simulink model "TwoLinkPlanarRobotHybridControl_gen2nomfiles"  (Simulink 9.0)
settings: Solver=ode1  StartTime=0.0  StopTime=10.0  FixedStep=0.01  RelTol=1e-3  EnableMultiTasking=on
values from neighbouring files (symbols this model uses):
  m = [1 1]    [FurutaPendulum_Dynamics.m]    (also in Question_2.m = [m_1 m_2]; test_ForwardDynamics.m = [1 1 1]; test_TwoLinkPlanarRobotDynamics.m = [m1 m2]; test_TwoLinkPlanarRobotHybridControl.m = [m1 m2])
  N = 5    [createEllipsoid.m]
  s = tf('s')    [Current_loop_bode.m]    (also in Question_1.m = 15)
  X = cos(0:2*pi/n:2*pi)    [createCylinder.m]
  Y = sin(0:2*pi/n:2*pi)    [createCylinder.m]
undefined symbols (not defined in the file or in its folder): Z
libraries: sm_lib x13, nesl_utility x9, simulink x1
settings Model: Creator=leavesdown_admin  LastModifiedBy=leavesdown
settings DataIOCC: LimitDataPoints=on  SignalLoggingSaveFormat=ModelDataLogs
settings OptimizationCC: ExpressionDepthLimit=2147483647
settings DebuggingCC: SolverPrmCheckMsg=warning  FcnCallInpInsideContextMsg=warning  StateNameClashWarn=warning
settings GRTTargetCC: GeneratePreprocessorConditionals=Disable all
settings SimscapeCC: SimscapeNormalizeSystem=off
settings ConfigurationSet: Description=SimMechanics 2G

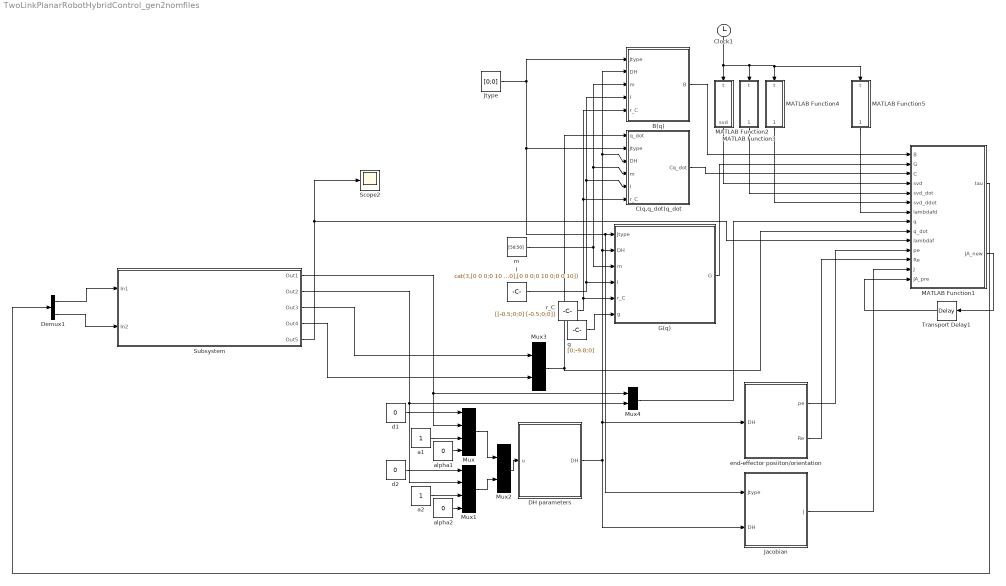
== system TwoLinkPlanarRobotHybridControl_gen2nomfiles ==
  B(q) : MATLAB Function  TreatAsAtomicUnit=on
  C(q,q_dot)q_dot : MATLAB Function  TreatAsAtomicUnit=on
  Clock1 : Clock
  DH parameters : MATLAB Function  TreatAsAtomicUnit=on
  Demux1 : Demux  Outputs=2
  G(q) : MATLAB Function  TreatAsAtomicUnit=on
  I : Constant  Value=cat(3,[0 0 0;0 10 0;0 0 10],[0 0 0;0 10 0;0 0 10])
  Jacobian : MATLAB Function  TreatAsAtomicUnit=on
  Jtype : Constant  Value=[0;0]
  MATLAB Function1 : MATLAB Function  TreatAsAtomicUnit=on
  MATLAB Function2 : MATLAB Function  TreatAsAtomicUnit=on
  MATLAB Function3 : MATLAB Function  TreatAsAtomicUnit=on
  MATLAB Function4 : MATLAB Function  TreatAsAtomicUnit=on
  MATLAB Function5 : MATLAB Function  TreatAsAtomicUnit=on
  Mux : Mux
  Mux1 : Mux
  Mux2 : Mux  Inputs=2
  Mux3 : Mux  Inputs=2
  Mux4 : Mux  Inputs=2
  Scope2 : Scope
  Subsystem : Subsystem
  Transport Delay1 : TransportDelay  DelayTime=0.01
  a1 : Constant
  a2 : Constant
  alpha1 : Constant  Value=0
  alpha2 : Constant  Value=0
  d1 : Constant  Value=0
  d2 : Constant  Value=0
  end-effector posiiton/orientation : MATLAB Function  TreatAsAtomicUnit=on
  g : Constant  Value=[0;-9.8;0]
  m : Constant  Value=[50;50]
  r_C : Constant  Value=[[-0.5;0;0] [-0.5;0;0]]
  wires:
  Subsystem/3(Out3) -> Mux3/1
  Demux1/2 -> Subsystem/2(In2)
  Subsystem/2(Out2) -> Mux4/2, Mux1/2
  Subsystem/4(Out4) -> Mux3/2
  Mux2/1 -> DH parameters/1(u)
  Mux3/1 -> MATLAB Function1/9(q_dot), C(q,q_dot)q_dot/1(q_dot)
  MATLAB Function4/1(svd_ddot) -> MATLAB Function1/6(svd_ddot)
  MATLAB Function3/1(svd_dot) -> MATLAB Function1/5(svd_dot)
  Mux1/1 -> Mux2/2
  m/1 -> B(q)/3(m), C(q,q_dot)q_dot/4(m), G(q)/3(m)
  Mux/1 -> Mux2/1
  MATLAB Function1/2(JA_new) -> Transport Delay1/1
  d1/1 -> Mux/1
  C(q,q_dot)q_dot/1(Cq_dot) -> MATLAB Function1/3(C)
  MATLAB Function2/1(svd) -> MATLAB Function1/4(svd)
  Jtype/1 -> B(q)/1(Jtype), C(q,q_dot)q_dot/2(Jtype), Jacobian/1(Jtype), G(q)/1(Jtype)
  alpha1/1 -> Mux/4
  G(q)/1(G) -> MATLAB Function1/2(G)
  a1/1 -> Mux/3
  alpha2/1 -> Mux1/4
  a2/1 -> Mux1/3
  r_C/1 -> B(q)/5(r_C), C(q,q_dot)q_dot/6(r_C), G(q)/5(r_C)
  Subsystem/1(Out1) -> Mux4/1, Mux/2
  B(q)/1(B) -> MATLAB Function1/1(B)
  Clock1/1 -> MATLAB Function5/1(t), MATLAB Function4/1(t), MATLAB Function3/1(t), MATLAB Function2/1(t)
  Demux1/1 -> Subsystem/1(In1)
  d2/1 -> Mux1/1
  g/1 -> G(q)/6(g)
  MATLAB Function1/1(tau) -> Demux1/1
  I/1 -> B(q)/4(I), C(q,q_dot)q_dot/5(I), G(q)/4(I)
  DH parameters/1(DH) -> Jacobian/2(DH), end-effector posiiton/orientation/1(DH), C(q,q_dot)q_dot/3(DH), B(q)/2(DH), G(q)/2(DH)
  Mux4/1 -> MATLAB Function1/8(q)
  Subsystem/5(Out5) -> MATLAB Function1/10(lambdaf), Scope2/1
  MATLAB Function5/1(lambdafd) -> MATLAB Function1/7(lambdafd)
  Jacobian/1(J) -> MATLAB Function1/13(J)
  Transport Delay1/1 -> MATLAB Function1/14(JA_pre)
  end-effector posiiton/orientation/1(pe) -> MATLAB Function1/11(pe)
  end-effector posiiton/orientation/2(Re) -> MATLAB Function1/12(Re)

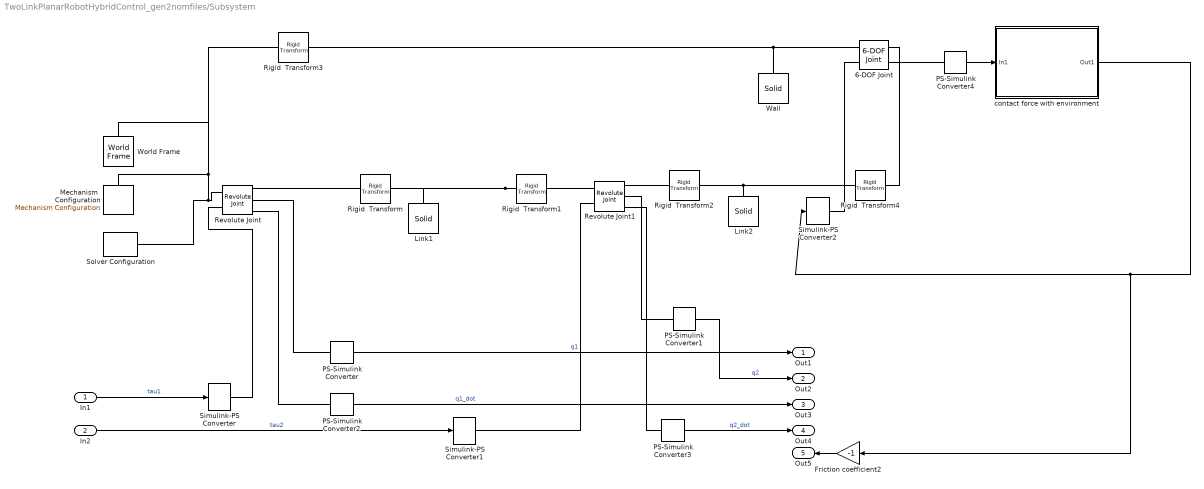
== system TwoLinkPlanarRobotHybridControl_gen2nomfiles/Subsystem ==
  In1 : Inport
  In2 : Inport  Port=2
  6-DOF Joint : sm_lib/Joints/6-DOF Joint  SenseConstraintForce=off  SenseConstraintForceX=off  SenseConstraintForceY=off  SenseConstraintForceZ=off  SenseConstraintTorque=off  SenseConstraintTorqueX=off  SenseConstraintTorqueY=off  SenseConstraintTorqueZ=off  SenseTotalForce=off  SenseTotalForceX=off  SenseTotalForceY=off  SenseTotalForceZ=off  SenseTotalTorque=off  SenseTotalTorqueX=off  SenseTotalTorqueY=off  SenseTotalTorqueZ=off  CompositeWrenchDir=FollowerOnBase  CompositeWrenchFrame=BaseFrame  PxEquilibriumPosition=0  PxEquilibriumPositionUnits=m  PxSpringStiffness=0  PxSpringStiffnessUnits=N/m  PxDampingCoefficient=0  PxDampingCoefficientUnits=N/(m/s)  PxTorqueActuationMode=NoTorque  PxMotionActuationMode=ComputedMotion  PxSensePosition=off  PxSenseVelocity=off  PxSenseAcceleration=off  PxSenseTorqueForce=off  PxPositionTargetSpecify=off  PxPositionTargetPriority=High  PxPositionTargetValue=0  PxPositionTargetValueUnits=m  PxVelocityTargetSpecify=off  PxVelocityTargetPriority=High  PxVelocityTargetValue=0  PxVelocityTargetValueUnits=m/s  PyEquilibriumPosition=0  PyEquilibriumPositionUnits=m  PySpringStiffness=0  PySpringStiffnessUnits=N/m  PyDampingCoefficient=0  PyDampingCoefficientUnits=N/(m/s)  PyTorqueActuationMode=InputTorque  PyMotionActuationMode=ComputedMotion  PySensePosition=on  PySenseVelocity=off  PySenseAcceleration=off  PySenseTorqueForce=off  PyPositionTargetSpecify=off  PyPositionTargetPriority=High  PyPositionTargetValue=0  PyPositionTargetValueUnits=m  PyVelocityTargetSpecify=off  PyVelocityTargetPriority=High  PyVelocityTargetValue=0  PyVelocityTargetValueUnits=m/s  PzEquilibriumPosition=0  PzEquilibriumPositionUnits=m  PzSpringStiffness=0  PzSpringStiffnessUnits=N/m  PzDampingCoefficient=0  PzDampingCoefficientUnits=N/(m/s)  PzTorqueActuationMode=NoTorque  PzMotionActuationMode=ComputedMotion  PzSensePosition=off  PzSenseVelocity=off  PzSenseAcceleration=off  PzSenseTorqueForce=off  PzPositionTargetSpecify=off  PzPositionTargetPriority=High  PzPositionTargetValue=0  PzPositionTargetValueUnits=m  PzVelocityTargetSpecify=off  PzVelocityTargetPriority=High  PzVelocityTargetValue=0  PzVelocityTargetValueUnits=m/s  SphDefPosRotationMethod=None  SphDefPosRotationAngleUnits=deg  SphDefPosRotationStandardAxis=+Z  SphDefPosRotationAngle=0  SphDefPosRotationArbitraryAxis=[0 0 1]  SphDefPosFollAlignAxisA=+X  SphDefPosBaseAlignAxisA=+Y  SphDefPosFollAlignAxisB=+Y  SphDefPosBaseAlignAxisB=+Z  SphDefPosRotationSequenceAxes=FollowerAxes  SphDefPosRotationSequence=XYX  SphDefPosRotationSequenceAngles=[0 0 0]  SphDefPosRotationSequenceAnglesUnits=deg  SphDefPosRotationMatrix=[1 0 0; 0 1 0; 0 0 1]  SphEqPosRotationMethod=None  SphEqPosRotationAngleUnits=deg  SphEqPosRotationStandardAxis=+Z  SphEqPosRotationAngle=0  SphEqPosRotationArbitraryAxis=[0 0 1]  SphEqPosFollAlignAxisA=+X  SphEqPosBaseAlignAxisA=+Y  SphEqPosFollAlignAxisB=+Y  SphEqPosBaseAlignAxisB=+Z  SphEqPosRotationSequenceAxes=FollowerAxes  SphEqPosRotationSequence=XYX  SphEqPosRotationSequenceAngles=[0 0 0]  SphEqPosRotationSequenceAnglesUnits=deg  SphEqPosRotationMatrix=[1 0 0; 0 1 0; 0 0 1]  SphSpringStiffness=0  SphSpringStiffnessUnits=N*m/deg  SphDampingCoefficient=0  SphDampingCoefficientUnits=N*m/(deg/s)  SphActuateTorqueX=off  SphActuateTorqueY=off  SphActuateTorqueZ=off  SphActuateTorque=off  SphTorqueActuationMode=NoTorque  SphMotionActuationMode=ComputedMotion  SphActuationFrame=BaseFrame  SphSensePosition=off  SphSenseVelocityX=off  SphSenseVelocityY=off  SphSenseVelocityZ=off  SphSenseVelocity=off  SphSenseAccelerationX=off  SphSenseAccelerationY=off  SphSenseAccelerationZ=off  SphSenseAcceleration=off  SphSenseTorqueX=off  SphSenseTorqueY=off  SphSenseTorqueZ=off  SphSenseTorqueForce=off  SphSensingFrame=BaseFrame  SphPositionTargetRotationMethod=None  SphPositionTargetRotationAngleUnits=deg  SphPositionTargetRotationStandardAxis=+Z  SphPositionTargetRotationAngle=0  SphPositionTargetRotationArbitraryAxis=[0 0 1]  SphPositionTargetFollAlignAxisA=+X  SphPositionTargetBaseAlignAxisA=+Y  SphPositionTargetFollAlignAxisB=+Y  SphPositionTargetBaseAlignAxisB=+Z  SphPositionTargetRotationSequenceAxes=FollowerAxes  SphPositionTargetRotationSequence=XYX  SphPositionTargetRotationSequenceAngles=[0 0 0]  SphPositionTargetRotationSequenceAnglesUnits=deg  SphPositionTargetRotationMatrix=[1 0 0; 0 1 0; 0 0 1]  SphPositionTargetSpecify=off  SphPositionTargetPriority=High  SphVelocityTargetValue=[0 0 0]  SphVelocityTargetValueUnits=deg/s  SphVelocityTargetSpecify=off  SphVelocityTargetPriority=High  SphVelocityTargetInFollowerFrame=on
  Friction coefficient2 : Gain  Gain=-1
  Link1 : sm_lib/Body Elements/Solid  InertiaType=Custom  Mass=50  MassUnits=kg  CenterOfMass=[0 0 0]  CenterOfMassUnits=m  MomentsOfInertia=[0 10 10]  MomentsOfInertiaUnits=kg*m^2  ProductsOfInertia=[0 0 0]  ProductsOfInertiaUnits=kg*m^2  DensityBased=on  Density=1000  DensityUnits=kg/(m^3)  DoExposeReferenceFrame=on  SerializedFrames=<Frames/>  GraphicType=FromGeometry  MarkerShape=Sphere  MarkerSize=10  MarkerSizeUnits=m  GraphicVisPropType=SimpleVisualProperties  GraphicDiffuseColor=[0.5 0.5 0.5]  GraphicSpecularColor=[0.5 0.5 0.5 1.0]  GraphicAmbientColor=[0.15 0.15 0.15 1.0]  GraphicEmissiveColor=[0.0 0.0 0.0 1.0]  GraphicShininess=75  GraphicOpacity=1.0  GeometryShape=Brick  RectangleSize=[1 1]  RectangleSizeUnits=m  BrickDimensions=[1 0.1 0.1]  BrickDimensionUnits=m  CylinderRadius=0.1  CylinderRadiusUnits=m  CylinderLength=1  CylinderLengthUnits=m  SphereRadius=1  SphereRadiusUnits=m  EllipsoidRadii=[1 1 1]  EllipsoidRadiiUnits=m  ExtrusionCrossSection=[1 1; -1 1; -1 -1; 1 -1]  ExtrusionCrossSectionUnits=m  ExtrusionLength=1  ExtrusionLengthUnits=m  PolygonNumSides=3  PolygonOuterRadius=1  PolygonOuterRadiusUnits=m  ExtGeomFileType=STEP  ExtGeomFileUnits=m  RevolutionCrossSection=[1 1; 1 -1; 2 -1; 2 1]  RevolutionCrossSectionUnits=m  RevolutionExtent=Full  RevolutionAngle=180  RevolutionAngleUnits=deg
  Link2 : sm_lib/Body Elements/Solid  InertiaType=Custom  Mass=50  MassUnits=kg  CenterOfMass=[0 0 0]  CenterOfMassUnits=m  MomentsOfInertia=[0 10 10]  MomentsOfInertiaUnits=kg*m^2  ProductsOfInertia=[0 0 0]  ProductsOfInertiaUnits=kg*m^2  DensityBased=on  Density=1000  DensityUnits=kg/(m^3)  DoExposeReferenceFrame=on  SerializedFrames=<Frames/>  GraphicType=FromGeometry  MarkerShape=Sphere  MarkerSize=10  MarkerSizeUnits=m  GraphicVisPropType=SimpleVisualProperties  GraphicDiffuseColor=[0.5 0.5 0.5]  GraphicSpecularColor=[0.5 0.5 0.5 1.0]  GraphicAmbientColor=[0.15 0.15 0.15 1.0]  GraphicEmissiveColor=[0.0 0.0 0.0 1.0]  GraphicShininess=75  GraphicOpacity=1.0  GeometryShape=Brick  RectangleSize=[1 1]  RectangleSizeUnits=m  BrickDimensions=[1 0.1 0.1]  BrickDimensionUnits=m  CylinderRadius=0.1  CylinderRadiusUnits=m  CylinderLength=1  CylinderLengthUnits=m  SphereRadius=1  SphereRadiusUnits=m  EllipsoidRadii=[1 1 1]  EllipsoidRadiiUnits=m  ExtrusionCrossSection=[1 1; -1 1; -1 -1; 1 -1]  ExtrusionCrossSectionUnits=m  ExtrusionLength=1  ExtrusionLengthUnits=m  PolygonNumSides=3  PolygonOuterRadius=1  PolygonOuterRadiusUnits=m  ExtGeomFileType=STEP  ExtGeomFileUnits=m  RevolutionCrossSection=[1 1; 1 -1; 2 -1; 2 1]  RevolutionCrossSectionUnits=m  RevolutionExtent=Full  RevolutionAngle=180  RevolutionAngleUnits=deg
  Mechanism  Configuration : sm_lib/Utilities/Mechanism Configuration  UniformGravity=Constant  GravityVector=[0 -9.81 0]  GravityUnits=m/s^2  LinearizationDelta=0.001
  PS-Simulink Converter{,1..4} (5 alike) : nesl_utility/PS-Simulink Converter  PhysicalDomain=network_engine_domain  SubClassName=ps_output  LeftPortType=input  RightPortType=output  PseudoPeriodic=off  Frequencies=[]  Unit=1  AffineConversion=off
  Revolute Joint : sm_lib/Joints/Revolute Joint  SenseConstraintForce=off  SenseConstraintForceX=off  SenseConstraintForceY=off  SenseConstraintForceZ=off  SenseConstraintTorque=off  SenseConstraintTorqueX=off  SenseConstraintTorqueY=off  SenseConstraintTorqueZ=off  SenseTotalForce=off  SenseTotalForceX=off  SenseTotalForceY=off  SenseTotalForceZ=off  SenseTotalTorque=off  SenseTotalTorqueX=off  SenseTotalTorqueY=off  SenseTotalTorqueZ=off  CompositeWrenchDir=FollowerOnBase  CompositeWrenchFrame=BaseFrame  EquilibriumPosition=0  EquilibriumPositionUnits=deg  SpringStiffness=0  SpringStiffnessUnits=N*m/deg  DampingCoefficient=50  DampingCoefficientUnits=N*m/(rad/s)  TorqueActuationMode=InputTorque  MotionActuationMode=ComputedMotion  SensePosition=on  SenseVelocity=on  SenseAcceleration=off  SenseTorqueForce=off  PositionTargetSpecify=on  PositionTargetPriority=High  PositionTargetValue=0  PositionTargetValueUnits=rad  VelocityTargetSpecify=off  VelocityTargetPriority=High  VelocityTargetValue=0  VelocityTargetValueUnits=deg/s
  Revolute Joint1 : sm_lib/Joints/Revolute Joint  SenseConstraintForce=off  SenseConstraintForceX=off  SenseConstraintForceY=off  SenseConstraintForceZ=off  SenseConstraintTorque=off  SenseConstraintTorqueX=off  SenseConstraintTorqueY=off  SenseConstraintTorqueZ=off  SenseTotalForce=off  SenseTotalForceX=off  SenseTotalForceY=off  SenseTotalForceZ=off  SenseTotalTorque=off  SenseTotalTorqueX=off  SenseTotalTorqueY=off  SenseTotalTorqueZ=off  CompositeWrenchDir=FollowerOnBase  CompositeWrenchFrame=BaseFrame  EquilibriumPosition=0  EquilibriumPositionUnits=deg  SpringStiffness=0  SpringStiffnessUnits=N*m/deg  DampingCoefficient=50  DampingCoefficientUnits=N*m/(rad/s)  TorqueActuationMode=InputTorque  MotionActuationMode=ComputedMotion  SensePosition=on  SenseVelocity=on  SenseAcceleration=off  SenseTorqueForce=off  PositionTargetSpecify=on  PositionTargetPriority=High  PositionTargetValue=pi/2  PositionTargetValueUnits=rad  VelocityTargetSpecify=off  VelocityTargetPriority=High  VelocityTargetValue=0  VelocityTargetValueUnits=deg/s
  Rigid  Transform{,1..2,4} (4 alike) : sm_lib/Frames and Transforms/Rigid Transform  TranslationMethod=Cartesian  TranslationStandardOffset=0  TranslationLengthUnit=m  TranslationStandardAxis=+Z  TranslationCartesianOffset=[0.5 0 0]  TranslationROffset=0  TranslationROffsetUnits=m  TranslationZOffset=0  TranslationZOffsetUnits=m  TranslationThetaOffset=0  TranslationThetaOffsetUnits=deg  RotationMethod=None  RotationAngleUnits=deg  RotationStandardAxis=+Z  RotationAngle=0  RotationArbitraryAxis=[0 0 1]  FollAlignAxisA=+X  BaseAlignAxisA=+Y  FollAlignAxisB=+Y  BaseAlignAxisB=+Z  RotationSequenceAxes=FollowerAxes  RotationSequence=XYX  RotationSequenceAngles=[0 0 0]  RotationSequenceAnglesUnits=deg  RotationMatrix=[1 0 0; 0 1 0; 0 0 1]
  Rigid  Transform3 : sm_lib/Frames and Transforms/Rigid Transform  TranslationMethod=Cartesian  TranslationStandardOffset=0  TranslationLengthUnit=m  TranslationStandardAxis=+Z  TranslationCartesianOffset=[1 1 0]  TranslationROffset=0  TranslationROffsetUnits=m  TranslationZOffset=0  TranslationZOffsetUnits=m  TranslationThetaOffset=0  TranslationThetaOffsetUnits=deg  RotationMethod=StandardAxis  RotationAngleUnits=rad  RotationStandardAxis=+Z  RotationAngle=-pi/4  RotationArbitraryAxis=[0 0 1]  FollAlignAxisA=+X  BaseAlignAxisA=+Y  FollAlignAxisB=+Y  BaseAlignAxisB=+Z  RotationSequenceAxes=FollowerAxes  RotationSequence=XYX  RotationSequenceAngles=[0 0 0]  RotationSequenceAnglesUnits=deg  RotationMatrix=[1 0 0; 0 1 0; 0 0 1]
  Simulink-PS Converter : nesl_utility/Simulink-PS Converter  PhysicalDomain=network_engine_domain  SubClassName=ps_input  LeftPortType=input  RightPortType=output  PseudoPeriodic=off  Frequencies=[]  NoiseDistribution=none  NoiseParameters=[]  Unit=1  AffineConversion=off  FilteringAndDerivatives=zero  SimscapeFilterOrder=1  InputFilterTimeConstant=.001  UdotUserProvided=[]
  Simulink-PS Converter1 : nesl_utility/Simulink-PS Converter  PhysicalDomain=network_engine_domain  SubClassName=ps_input  LeftPortType=input  RightPortType=output  PseudoPeriodic=off  Frequencies=[]  NoiseDistribution=none  NoiseParameters=[]  Unit=1  AffineConversion=off  FilteringAndDerivatives=zero  SimscapeFilterOrder=1  InputFilterTimeConstant=.001  UdotUserProvided=[]
  Simulink-PS Converter2 : nesl_utility/Simulink-PS Converter  PhysicalDomain=network_engine_domain  SubClassName=ps_input  LeftPortType=input  RightPortType=output  PseudoPeriodic=off  Frequencies=[]  NoiseDistribution=none  NoiseParameters=[]  Unit=1  AffineConversion=off  FilteringAndDerivatives=zero  SimscapeFilterOrder=1  InputFilterTimeConstant=.001  UdotUserProvided=[]
  Solver Configuration : nesl_utility/Solver Configuration  PhysicalDomain=network_engine_domain  SubClassName=solver  LeftPortType=input  RightPortType=generic  Accelerate=off  Tones=[]  Harmonics=[]  SimulateNoise=off  Profile=off  UseLocalSampling=off  EnableSwitchedLinearOptims=on  FrequencyDomain=off  UseCCode=off  RelTol=0.001  AbsTol=1e-06  MinStep=1e-09  ToWorkspace=off  RevertToSquareIcSolve=off  NumHomotopyIterations=100  PhasorMode=off  PhasorModeNumHarmonics=1  DoDC=off  ResidualTolerance=1e-9  UseLocalSolver=off  LocalSolverChoice=NE_BACKWARD_EULER_ADVANCER  LocalSolverSampleTime=.01  DoFixedCost=off  MaxNonlinIter=3  MaxModeIter=2  LinearAlgebra=Sparse  DelaysMemoryBudget=1024  AutomaticFiltering=on  FilteringTimeConstant=0.001
  Wall : sm_lib/Body Elements/Solid  InertiaType=Custom  Mass=50  MassUnits=kg  CenterOfMass=[0 0 0]  CenterOfMassUnits=m  MomentsOfInertia=[0 10 10]  MomentsOfInertiaUnits=kg*m^2  ProductsOfInertia=[0 0 0]  ProductsOfInertiaUnits=kg*m^2  DensityBased=on  Density=1000  DensityUnits=kg/(m^3)  DoExposeReferenceFrame=on  SerializedFrames=<Frames/>  GraphicType=FromGeometry  MarkerShape=Sphere  MarkerSize=10  MarkerSizeUnits=m  GraphicVisPropType=SimpleVisualProperties  GraphicDiffuseColor=[0.5 0.5 0.5]  GraphicSpecularColor=[0.5 0.5 0.5 1.0]  GraphicAmbientColor=[0.15 0.15 0.15 1.0]  GraphicEmissiveColor=[0.0 0.0 0.0 1.0]  GraphicShininess=75  GraphicOpacity=1.0  GeometryShape=Brick  RectangleSize=[1 1]  RectangleSizeUnits=m  BrickDimensions=[2 0.1 2]  BrickDimensionUnits=m  CylinderRadius=0.1  CylinderRadiusUnits=m  CylinderLength=1  CylinderLengthUnits=m  SphereRadius=1  SphereRadiusUnits=m  EllipsoidRadii=[1 1 1]  EllipsoidRadiiUnits=m  ExtrusionCrossSection=[1 1; -1 1; -1 -1; 1 -1]  ExtrusionCrossSectionUnits=m  ExtrusionLength=1  ExtrusionLengthUnits=m  PolygonNumSides=3  PolygonOuterRadius=1  PolygonOuterRadiusUnits=m  ExtGeomFileType=STEP  ExtGeomFileUnits=m  RevolutionCrossSection=[1 1; 1 -1; 2 -1; 2 1]  RevolutionCrossSectionUnits=m  RevolutionExtent=Full  RevolutionAngle=180  RevolutionAngleUnits=deg
  World Frame : sm_lib/Frames and Transforms/World Frame
  contact force with environment : Subsystem
  Out1 : Outport
  Out2 : Outport  Port=2
  Out3 : Outport  Port=3
  Out4 : Outport  Port=4
  Out5 : Outport  Port=5
  wires:
  PS-Simulink Converter1/1 -> Out2/1  "q2"
  PS-Simulink Converter/1 -> Out1/1  "q1"
  PS-Simulink Converter3/1 -> Out4/1  "q2_dot"
  In2/1 -> Simulink-PS Converter1/1  "tau2"
  PS-Simulink Converter2/1 -> Out3/1  "q1_dot"
  In1/1 -> Simulink-PS Converter/1  "tau1"
  contact force with environment/1(Out1) -> Simulink-PS Converter2/1, Friction coefficient2/1
  PS-Simulink Converter4/1 -> contact force with environment/1(In1)
  Friction coefficient2/1 -> Out5/1
  connections:
  Rigid  Transform1/LConn1 -- Link1/RConn1 -- Rigid  Transform/RConn1
  Solver Configuration/RConn1 -- Rigid  Transform3/LConn1 -- World Frame/RConn1 -- Mechanism  Configuration/RConn1 -- Revolute Joint/LConn1
  Simulink-PS Converter/RConn1 -- Revolute Joint/LConn2
  PS-Simulink Converter3/LConn1 -- Revolute Joint1/RConn3
  Rigid  Transform/LConn1 -- Revolute Joint/RConn1
  Revolute Joint/RConn2 -- PS-Simulink Converter/LConn1
  Rigid  Transform1/RConn1 -- Revolute Joint1/LConn1
  Simulink-PS Converter1/RConn1 -- Revolute Joint1/LConn2
  Rigid  Transform2/RConn1 -- Rigid  Transform4/LConn1 -- Link2/RConn1
  Revolute Joint1/RConn1 -- Rigid  Transform2/LConn1
  Revolute Joint1/RConn2 -- PS-Simulink Converter1/LConn1
  Revolute Joint/RConn3 -- PS-Simulink Converter2/LConn1
  Rigid  Transform3/RConn1 -- 6-DOF Joint/LConn1 -- Wall/RConn1
  6-DOF Joint/RConn2 -- PS-Simulink Converter4/LConn1
  Rigid  Transform4/RConn1 -- 6-DOF Joint/RConn1
  Simulink-PS Converter2/RConn1 -- 6-DOF Joint/LConn2

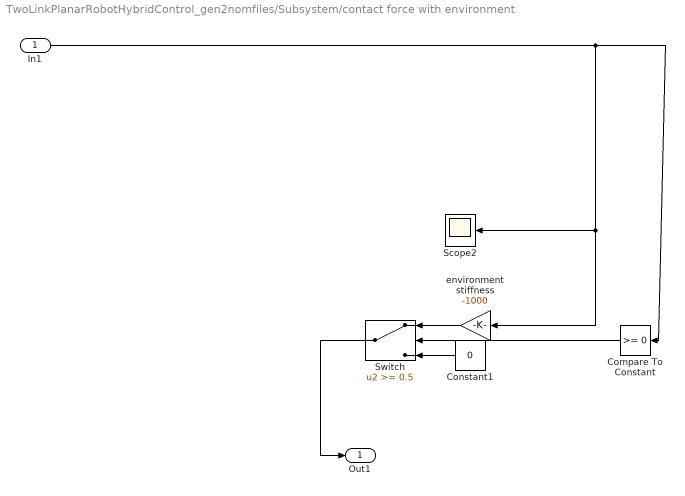
== system TwoLinkPlanarRobotHybridControl_gen2nomfiles/Subsystem/contact force with environment ==
  In1 : Inport
  Compare To Constant : simulink/Logic and Bit Operations/Compare To Constant  relop=>=  const=0  OutDataTypeStr=uint8
  Constant1 : Constant  Value=0
  Scope2 : Scope
  Switch : Switch  Threshold=0.5
  environment stiffness : Gain  Gain=-1000
  Out1 : Outport
  wires:
  In1/1 -> Compare To Constant/1, environment stiffness/1, Scope2/1
  Compare To Constant/1 -> Switch/2
  environment stiffness/1 -> Switch/1
  Constant1/1 -> Switch/3
  Switch/1 -> Out1/1

== matlab function B(q) ==
  data: Jtype input double; B output double; DH input double; m input double; I input double; r_C input double
function B = fcn(Jtype,DH,m,I,r_C)
coder.extrinsic('Newton_Euler_Iteration');
n=length(m);%number of joints

B=zeros(n,n);
for i=1:n
    q_ddot_temp=[0;0];
    q_ddot_temp(i)=1;
    B(:,i) = Newton_Euler_Iteration(DH, m, I, r_C, Jtype, zeros(n,1), q_ddot_temp,zeros(3,1));
end

== matlab function C(q,q_dot)q_dot ==
  data: q_dot input double; Jtype input double; Cq_dot output double; DH input double; m input double; I input double; r_C input double
function Cq_dot = fcn(q_dot,Jtype,DH,m,I,r_C)
coder.extrinsic('Newton_Euler_Iteration');
n=length(m);%number of joints
Cq_dot=zeros(n,1);
Cq_dot=Newton_Euler_Iteration(DH, m, I, r_C, Jtype, q_dot, zeros(n,1), zeros(3,1));%compute C(q,\dot{q})\dot{q}

== matlab function G(q) ==
  data: Jtype input double; G output double; DH input double; m input double; I input double; r_C input double; g input double
function G = fcn(Jtype,DH,m,I,r_C,g)
coder.extrinsic('Newton_Euler_Iteration');
n=length(m);%number of joints
G=zeros(n,1);
G=Newton_Euler_Iteration(DH, m, I, r_C, Jtype, zeros(n,1), zeros(n,1), g);%compute C(q,\dot{q})\dot{q}

== matlab function DH parameters ==
  data: DH output double; u input double
function DH = fcn(u)
temp=reshape(u,4,length(u)/4);
DH=temp;

== matlab function MATLAB Function1 ==
  data: tau output double; B input double; G input double; C input double; svd input double; svd_dot input double; svd_ddot input double; lambdafd input double; q input double; q_dot input double; lambdaf input double; pe input double; Re input double; J input double; JA_new output double; JA_pre input double
function [tau,JA_new] = fcn(B,G,C,svd,svd_dot,svd_ddot,lambdafd,q,q_dot,lambdaf,pe,Re,J,JA_pre)
%size initialization
tau=zeros(2,1);
temp=zeros(2,1);

Sf=[cos(pi/4);sin(pi/4)];
Sv=[-sin(pi/4);cos(pi/4)];
JA_new=J(1:2,:);
dt=0.01;
JA_dot=(JA_new-JA_pre)./dt;%calculate the derivative of JA
Bm=50;Dm=400;Km=10;
temp=[Sf Sv]'*[pe(1);pe(2)];
sf=temp(1);sv=temp(2);
temp=[Sf Sv]'*JA_new*q_dot;
sf_dot=temp(1);sv_dot=temp(2);
sfc=sqrt(2);
lambdav=0;%friction force in unconstrained direction is zero

%position control law in unconstrained direction
ev=sv-svd;
ev_dot=sv_dot-svd_dot;
Kp=25;Kd=5;
av=svd_ddot-Kp*ev-Kd*ev_dot;
    
%direct force control in constrained direction
k_hat=1000;%estimation of contact stiffness k
%calculate the estimate of velocity in the constrained direction
%(lambdaf_dot)
if sf<sfc
    lambdaf_dot_hat=0;
else
    lambdaf_dot_hat=k_hat*sf_dot;
end
kp=100;kd=20;
af=-kp/k_hat*(lambdaf-lambdafd)-kd/k_hat*lambdaf_dot_hat;

    
% or,  impedance control in constrained direction
%     Mm=50;Dm=400;Km=10;
%     sfd=sfc+lambdafd/Km;
%     af=1/Mm*(-Dm*(sf_dot)-Km*(sf-sfd)-lambdaf);

kv=[50;50];%define viscous friction constants
tau=G+C+kv.*q_dot+JA_new'*(Sf*lambdaf+Sv*lambdav)+B*JA_new'*inv(JA_new*JA_new'+0.01.*eye(2))*(-JA_dot*q_dot+Sf*af+Sv*av);

== matlab function MATLAB Function2 ==
  data: t input double; svd output double
function svd = fcn(t)

svd = 0.5*sin(2*pi/2*t);

== matlab function MATLAB Function3 ==
  data: t input double; svd_dot output double
function svd_dot = fcn(t)

svd_dot = 0.5*2*pi/2*cos(2*pi/2*t);

== matlab function MATLAB Function4 ==
  data: t input double; svd_ddot output double
function svd_ddot = fcn(t)

svd_ddot = -0.5*(2*pi/2)^2*sin(2*pi/2*t);

== matlab function MATLAB Function5 ==
  data: t input double; lambdafd output double
function lambdafd = fcn(t)

lambdafd = 20; %desired contact force 20N

== matlab function end-effector posiiton//orientation ==
  data: pe output double; DH input double; Re output double
function [pe,Re] = fcn(DH)
coder.extrinsic('Forward_Kinematics');
Re=zeros(3,3);pe=zeros(3,1);
n=length(DH(1,:));%number of joints

A_lump=zeros(4,4,n);
A_lump = Forward_Kinematics(DH);
Ae=A_lump(:,:,n);
Re=Ae(1:3,1:3);
pe=Ae(1:3,4);

== matlab function Jacobian ==
  data: Jtype input double; J output double; DH input double
function J = fcn(Jtype,DH)
coder.extrinsic('Jacobian');
J = zeros(6,length(DH(1,:)));
J = Jacobian(DH,Jtype);
